simulink model "arduinowifi_udp_hostsend"  (R2017b)
settings: Solver=ode45  StartTime=0.0  StopTime=inf  RelTol=1e-3  EnableMultiTasking=on
libraries: xpcseriallib x1, svdutilitieslib x1, instrumentlib x1
settings Model: Creator=smohan  LastModifiedBy=admin
settings DataIOCC: LimitDataPoints=on  SaveFormat=Array
settings OptimizationCC: ExpressionDepthLimit=2147483647  LifeSpan=inf
settings DebuggingCC: UnderspecifiedInitializationDetection=Classic  MergeDetectMultiDrivingBlocksExec=none  AllowSymbolicDim=off  StateNameClashWarn=warning  SFUnexpectedBacktrackingDiag=warning  SFNoUnconditionalDefaultTransitionDiag=warning  SFExecutionAtInitializationDiag=none
settings HardwareCC: ProdBitPerPointer=32  ProdBitPerSizeT=32  ProdBitPerPtrDiffT=32  ProdLargestAtomicFloat=None  ProdIntDivRoundTo=Undefined  ProdEndianess=Unspecified  ProdWordSize=32  ProdHWDeviceType=32-bit Generic
settings ModelReferenceCC: PropagateSignalLabelsOutOfModel=off
settings CodeAppCC: StateflowObjectComments=on
settings GRTTargetCC: TargetLangStandard=C89/C90 (ANSI)  GeneratePreprocessorConditionals=Disable all
settings ConfigComp: CovMetricSettings=dw  CovHtmlReporting=on  CovSaveCumulativeToWorkspaceVar=on  CovSaveSingleToWorkspaceVar=on  CovExternalEMLEnable=off

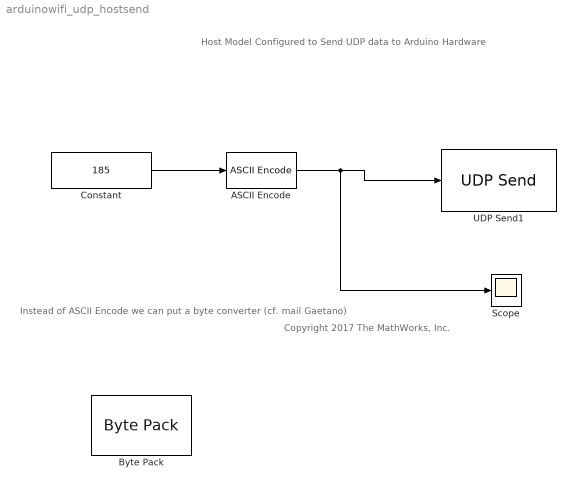
== system arduinowifi_udp_hostsend ==
  note: Copyright 2017 The MathWorks, Inc.
  note: Host Model Configured to Send
      | UDP data to Arduino Hardware
  note: Instead of ASCII Encode we can put a byte converter (cf. mail Gaetano)
  "ASCII Encode " : xpcseriallib/ASCII Encode   format=%d\r  nvars=1  maxlength=128  vartypes={ 'double' }
      settings: SourceProductName=Simulink Real-Time  SourceProductBaseCode=XP
  Byte Pack : svdutilitieslib/Byte Pack  datatypes={'uint8'}  byteAlign=1  blockPlatform=arduinoert
      settings: SourceProductName=Simulink Support Package for Arduino Hardware  SourceProductBaseCode=ARDUINO
  Constant : Constant  Value=185  OutDataTypeStr=double  SampleTime=5  LockScale=on
  Scope : Scope
  UDP Send1 : instrumentlib/UDP Send  Host=192.168.4.1  Port=333  LocalPort=-1  EnableBlockingMode=on  ByteOrder=LittleEndian
      settings: SourceProductName=Instrument Control Toolbox
  wires:
  Constant/1 -> "ASCII Encode "/1
  "ASCII Encode "/1 -> Scope/1, UDP Send1/1
